simulink model "ex3_b"  (R2020a)
settings: Solver=VariableStepAuto  StartTime=0.0  StopTime=10.0  RelTol=1e-3
settings Model: Creator=Tomo  LastModifiedBy=Tomo

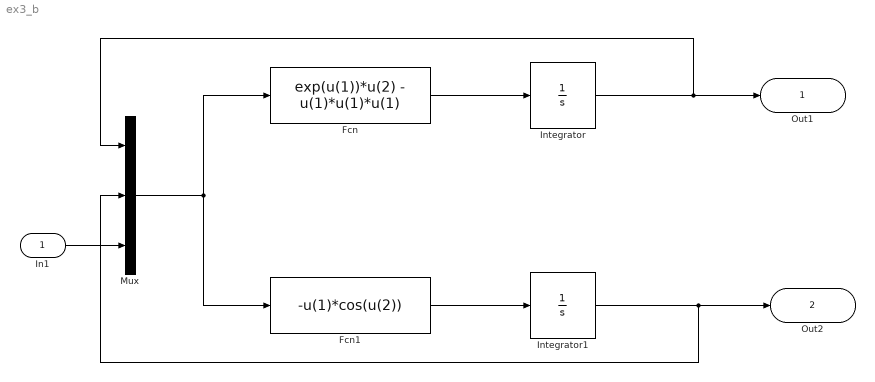
== system ex3_b ==
  In1 : Inport
  Fcn : Fcn  Expr=exp(u(1))*u(2) - u(1)*u(1)*u(1)
  Fcn1 : Fcn  Expr=-u(1)*cos(u(2))
  Integrator : Integrator
  Integrator1 : Integrator
  Mux : Mux  Inputs=3
  Out1 : Outport
  Out2 : Outport  Port=2
  wires:
  Fcn/1 -> Integrator/1
  Integrator/1 -> Mux/1, Out1/1
  Integrator1/1 -> Out2/1, Mux/2
  Fcn1/1 -> Integrator1/1
  Mux/1 -> Fcn/1, Fcn1/1
  In1/1 -> Mux/3
